simulink model "SMC_final"  (R2022b)
settings: Solver=ode14x  StartTime=0.0  StopTime=50  FixedStep=0.0002  RelTol=1e-3
undefined symbols (not defined in the file): g, I_xx, I_yy, I_zz, K_k_phi, K_k_psi, K_k_theta, K_k_x, K_k_y, K_k_z, lambda_phi, lambda_psi, lambda_theta, lambda_x, lambda_y, lambda_z, m, Psi_ref, X_ref, Y_ref, Z_ref
libraries: slpidlib x3
settings Model: Creator=User  LastModifiedBy=User
settings SolverCC: AlgebraicLoopSolver=TrustRegion
settings RTWCC: DLArmComputeVersion=19.05

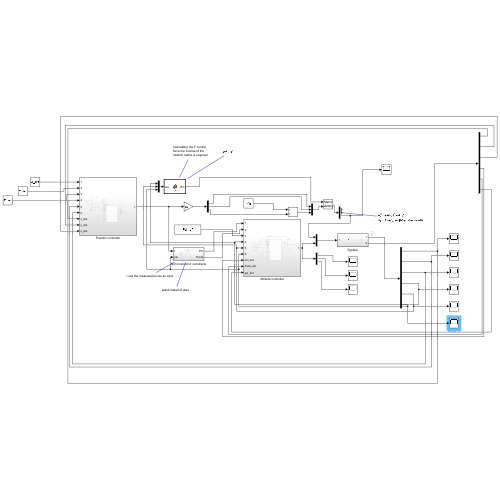
[thumbnail: Simulink's stored preview of the top-level diagram]
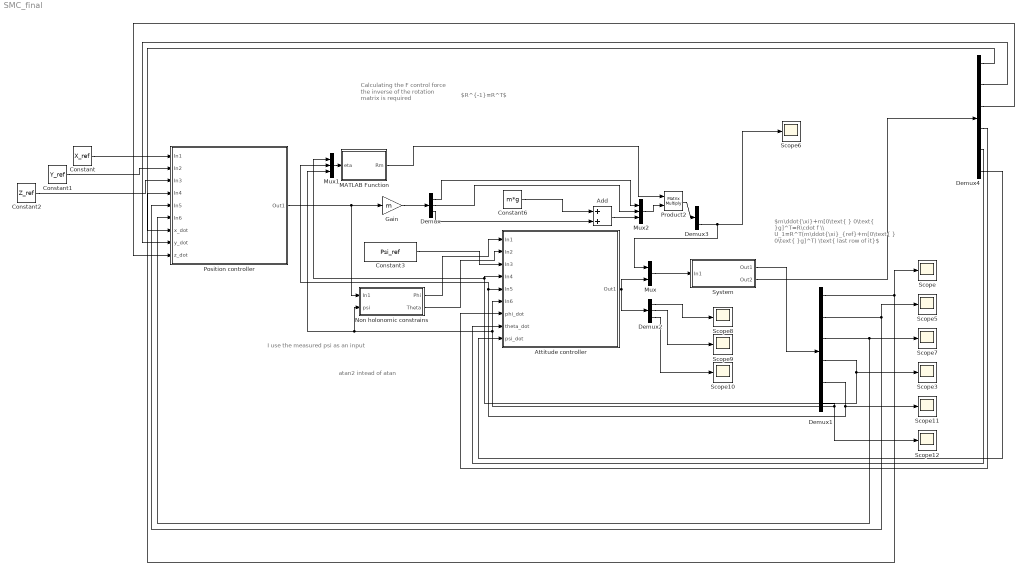
== system SMC_final ==
  note: $R^{-1}=R^T$
  note: $m\ddot{\xi}+m[0\text{ } 0\text{ }g]^T=R\cdot f \\ U_1=R^T(m\ddot{\xi}_{ref}+m[0\text{ } 0\text{ }g]^T) \text{ last row of it}$
  note: atan2 intead of atan
  note: Calculating the F control force the inverse of the rotation matrix is required
  note: I use the measured psi as an input
  Add : Sum
  Attitude controller : Subsystem
  Constant : Constant  Value=X_ref
  Constant1 : Constant  Value=Y_ref
  Constant2 : Constant  Value=Z_ref
  Constant3 : Constant  Value=Psi_ref
  Constant6 : Constant  Value=m*g
  Demux : Demux  Outputs=3
  Demux1 : Demux  Outputs=6
  Demux2 : Demux  Outputs=3
  Demux3 : Demux  Outputs=3
  Demux4 : Demux  Outputs=6
  Gain : Gain  Gain=m
  MATLAB Function : MATLAB Function  TreatAsAtomicUnit=on
  Mux : Mux  Inputs=2
  Mux1 : Mux  Inputs=3
  Mux2 : Mux  Inputs=3
  Non holonomic constrains : Subsystem
  Position controller : Subsystem
  Product2 : Product  Multiplication=Matrix(*)
  Scope{,3,5..12} (10 alike) : Scope
  System : Subsystem
  wires:
  System/1(Out1) -> Demux1/1
  Demux1/4 -> Scope3/1, Mux1/1, Attitude controller/4(In4)
  Demux1/1 -> Scope/1, Position controller/4(In4)
  Demux1/2 -> Scope5/1, Position controller/5(In5)
  Demux1/3 -> Scope7/1, Position controller/6(In6)
  Position controller/1(Out1) -> Non holonomic constrains/1(In1), Gain/1
  Non holonomic constrains/1(Phi) -> Attitude controller/1(In1)
  Non holonomic constrains/2(Theta) -> Attitude controller/2(In2)
  Demux1/5 -> Mux1/2, Attitude controller/5(In5), Scope11/1
  Demux1/6 -> Scope12/1, Non holonomic constrains/2(psi), Mux1/3, Attitude controller/6(In6)
  Attitude controller/1(Out1) -> Mux/2, Demux2/1
  Mux/1 -> System/1(In1)
  Demux/1 -> Mux2/1
  Demux/2 -> Mux2/2
  Demux2/1 -> Scope8/1
  Demux2/2 -> Scope9/1
  Demux2/3 -> Scope10/1
  Constant3/1 -> Attitude controller/3(In3)
  Demux/3 -> Add/2
  Mux1/1 -> MATLAB Function/1(eta)
  Add/1 -> Mux2/3
  MATLAB Function/1(Rm) -> Product2/1
  Mux2/1 -> Product2/2
  Product2/1 -> Demux3/1
  Demux3/3 -> Mux/1, Scope6/1
  Gain/1 -> Demux/1
  Constant/1 -> Position controller/1(In1)
  Constant1/1 -> Position controller/2(In2)
  Constant2/1 -> Position controller/3(In3)
  Constant6/1 -> Add/1
  System/2(Out2) -> Demux4/1
  Demux4/1 -> Position controller/7(x_dot)
  Demux4/2 -> Position controller/8(y_dot)
  Demux4/3 -> Position controller/9(z_dot)
  Demux4/4 -> Attitude controller/7(phi_dot)
  Demux4/5 -> Attitude controller/8(theta_dot)
  Demux4/6 -> Attitude controller/9(psi_dot)

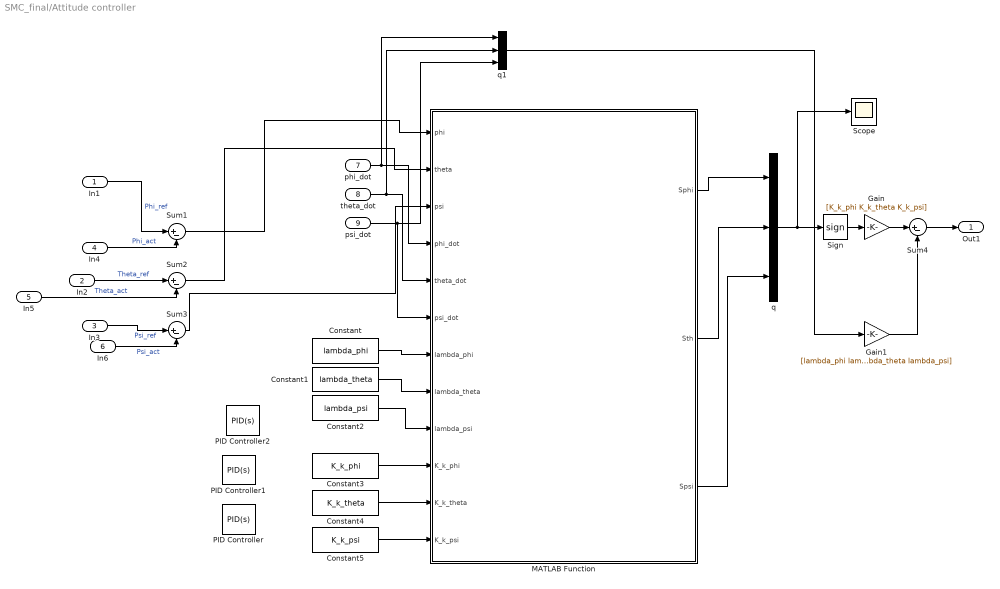
== system SMC_final/Attitude controller ==
  In1 : Inport
  In2 : Inport  Port=2
  In3 : Inport  Port=3
  In4 : Inport  Port=4
  In5 : Inport  Port=5
  In6 : Inport  Port=6
  phi_dot : Inport  Port=7
  theta_dot : Inport  Port=8
  psi_dot : Inport  Port=9
  Constant : Constant  Value=lambda_phi
  Constant1 : Constant  Value=lambda_theta
  Constant2 : Constant  Value=lambda_psi
  Constant3 : Constant  Value=K_k_phi
  Constant4 : Constant  Value=K_k_theta
  Constant5 : Constant  Value=K_k_psi
  Gain : Gain  Gain=[K_k_phi K_k_theta K_k_psi]
  Gain1 : Gain  Gain=[lambda_phi lambda_theta lambda_psi]
  MATLAB Function : MATLAB Function  TreatAsAtomicUnit=on
  PID Controller : slpidlib/PID Controller  Controller=PID  Form=Parallel  TimeDomain=Continuous-time  UseExternalTs=off  SampleTime=-1  IntegratorMethod=Forward Euler  FilterMethod=Forward Euler  ControllerParametersSource=internal  P=0.1  I=0  UseKiTs=off  D=0.05  N=100  UseFilter=on  TunerSelectOption=Transfer Function Based (PID Tuner App)  InitialConditionSource=internal  InitialConditionForIntegrator=0  InitialConditionForFilter=0  DifferentiatorICPrevScaledInput=0  ExternalReset=none  TrackingMode=off  Kt=1  LimitOutput=off  SatLimitsSource=internal  UpperSaturationLimit=inf  LowerSaturationLimit=-inf  LinearizeAsGain=on  AntiWindupMode=none  Kb=1  LimitIntegrator=off  UpperIntegratorSaturationLimit=inf  LowerIntegratorSaturationLimit=-inf  POutMin=[]  POutMax=[]  IOutMin=[]  IOutMax=[]  DOutMin=[]  DOutMax=[]  NOutMin=[]  NOutMax=[]  SumOutMin=[]  SumOutMax=[]  SaturationOutMin=[]  SaturationOutMax=[]  PParamMin=[]  PParamMax=[]  IParamMin=[]  IParamMax=[]  DParamMin=[]  DParamMax=[]  NParamMin=[]  NParamMax=[]  KbParamMin=[]  KbParamMax=[]  KtParamMin=[]  KtParamMax=[]  KbOutMin=[]  KbOutMax=[]  KtOutMin=[]  KtOutMax=[]  IntegratorOutMin=[]  IntegratorOutMax=[]  FilterOutMin=[]  FilterOutMax=[]  SumI1OutMin=[]  SumI1OutMax=[]  SumI2OutMin=[]  SumI2OutMax=[]  SumI3OutMin=[]  SumI3OutMax=[]  SumI4OutMin=[]  SumI4OutMax=[]  SumDOutMin=[]  SumDOutMax=[]  DifferentiatorOutMin=[]  DifferentiatorOutMax=[]  FilterDiffOutCoefMin=[]  FilterDiffOutCoefMax=[]  ReciprocalOutMin=[]  ReciprocalOutMax=[]  SumDenOutMin=[]  SumDenOutMax=[]  SumNumOutMin=[]  SumNumOutMax=[]  DivideOutMin=[]  DivideOutMax=[]  UdiffTsProdOutMin=[]  UdiffTsProdOutMax=[]  NTsProdOutMin=[]  NTsProdOutMax=[]  UintegralTsProdOutMin=[]  UintegralTsProdOutMax=[]  UngainTsProdOutMin=[]  UngainTsProdOutMax=[]  ClampingZeroOutDataTypeStr=Inherit: Inherit via back propagation  ClampingZeroOutMin=[]  ClampingZeroOutMax=[]  FilterDenConstantOutDataTypeStr=Inherit: Inherit via back propagation  FilterDenConstantOutMin=[]  FilterDenConstantOutMax=[]  PCopyOutDataTypeStr=Inherit: Inherit via back propagation  PCopyOutMin=[]  PCopyOutMax=[]  NCopyOutDataTypeStr=Inherit: Inherit via back propagation  NCopyOutMin=[]  NCopyOutMax=[]  IntegratorContinuousStateAttributes=''  IntegratorStateMustResolveToSignalObject=off  IntegratorRTWStateStorageClass=Auto  FilterContinuousStateAttributes=''  FilterStateMustResolveToSignalObject=off  FilterRTWStateStorageClass=Auto  ParallelPVariant=InternalParameters  IdealPVariant=Disabled  IVariant=InternalParameters  DVariant=InternalParameters  IntegratorVariant=Continuous  SatVariant=Disabled  AWVariant=Passthrough  PCopyVariant=Disabled  TRVariant=Disabled  FdbkBlocksVariant=Forward  IdealPFdbkVariant=Disabled  SatFdbkVariant=Disabled  DerivativeFilterVariant=ContFilter  NVariant=InternalParameters  NCopyVariant=Disabled  FilterICVariant=InternalICsFilter  IntegratorICVariant=InternalICs  ExternalResetVariant=Disabled  TRSumVariant=Passthrough  SumFdbkVariant=Disabled  SumVariant=Sum_PID  TsampFilterVariant=InternalTs  TsampNgainVariant=Passthrough  TsampIntegralVariant=Passthrough  ExternalSaturationOutDataTypeStr=Inherit: Same as second input
  PID Controller1 : slpidlib/PID Controller  Controller=PID  Form=Parallel  TimeDomain=Continuous-time  UseExternalTs=off  SampleTime=-1  IntegratorMethod=Forward Euler  FilterMethod=Forward Euler  ControllerParametersSource=internal  P=0.1  I=0  UseKiTs=off  D=0.05  N=100  UseFilter=on  TunerSelectOption=Transfer Function Based (PID Tuner App)  InitialConditionSource=internal  InitialConditionForIntegrator=0  InitialConditionForFilter=0  DifferentiatorICPrevScaledInput=0  ExternalReset=none  TrackingMode=off  Kt=1  LimitOutput=off  SatLimitsSource=internal  UpperSaturationLimit=inf  LowerSaturationLimit=-inf  LinearizeAsGain=on  AntiWindupMode=none  Kb=1  LimitIntegrator=off  UpperIntegratorSaturationLimit=inf  LowerIntegratorSaturationLimit=-inf  POutMin=[]  POutMax=[]  IOutMin=[]  IOutMax=[]  DOutMin=[]  DOutMax=[]  NOutMin=[]  NOutMax=[]  SumOutMin=[]  SumOutMax=[]  SaturationOutMin=[]  SaturationOutMax=[]  PParamMin=[]  PParamMax=[]  IParamMin=[]  IParamMax=[]  DParamMin=[]  DParamMax=[]  NParamMin=[]  NParamMax=[]  KbParamMin=[]  KbParamMax=[]  KtParamMin=[]  KtParamMax=[]  KbOutMin=[]  KbOutMax=[]  KtOutMin=[]  KtOutMax=[]  IntegratorOutMin=[]  IntegratorOutMax=[]  FilterOutMin=[]  FilterOutMax=[]  SumI1OutMin=[]  SumI1OutMax=[]  SumI2OutMin=[]  SumI2OutMax=[]  SumI3OutMin=[]  SumI3OutMax=[]  SumI4OutMin=[]  SumI4OutMax=[]  SumDOutMin=[]  SumDOutMax=[]  DifferentiatorOutMin=[]  DifferentiatorOutMax=[]  FilterDiffOutCoefMin=[]  FilterDiffOutCoefMax=[]  ReciprocalOutMin=[]  ReciprocalOutMax=[]  SumDenOutMin=[]  SumDenOutMax=[]  SumNumOutMin=[]  SumNumOutMax=[]  DivideOutMin=[]  DivideOutMax=[]  UdiffTsProdOutMin=[]  UdiffTsProdOutMax=[]  NTsProdOutMin=[]  NTsProdOutMax=[]  UintegralTsProdOutMin=[]  UintegralTsProdOutMax=[]  UngainTsProdOutMin=[]  UngainTsProdOutMax=[]  ClampingZeroOutDataTypeStr=Inherit: Inherit via back propagation  ClampingZeroOutMin=[]  ClampingZeroOutMax=[]  FilterDenConstantOutDataTypeStr=Inherit: Inherit via back propagation  FilterDenConstantOutMin=[]  FilterDenConstantOutMax=[]  PCopyOutDataTypeStr=Inherit: Inherit via back propagation  PCopyOutMin=[]  PCopyOutMax=[]  NCopyOutDataTypeStr=Inherit: Inherit via back propagation  NCopyOutMin=[]  NCopyOutMax=[]  IntegratorContinuousStateAttributes=''  IntegratorStateMustResolveToSignalObject=off  IntegratorRTWStateStorageClass=Auto  FilterContinuousStateAttributes=''  FilterStateMustResolveToSignalObject=off  FilterRTWStateStorageClass=Auto  ParallelPVariant=InternalParameters  IdealPVariant=Disabled  IVariant=InternalParameters  DVariant=InternalParameters  IntegratorVariant=Continuous  SatVariant=Disabled  AWVariant=Passthrough  PCopyVariant=Disabled  TRVariant=Disabled  FdbkBlocksVariant=Forward  IdealPFdbkVariant=Disabled  SatFdbkVariant=Disabled  DerivativeFilterVariant=ContFilter  NVariant=InternalParameters  NCopyVariant=Disabled  FilterICVariant=InternalICsFilter  IntegratorICVariant=InternalICs  ExternalResetVariant=Disabled  TRSumVariant=Passthrough  SumFdbkVariant=Disabled  SumVariant=Sum_PID  TsampFilterVariant=InternalTs  TsampNgainVariant=Passthrough  TsampIntegralVariant=Passthrough  ExternalSaturationOutDataTypeStr=Inherit: Same as second input
  PID Controller2 : slpidlib/PID Controller  Controller=PID  Form=Parallel  TimeDomain=Continuous-time  UseExternalTs=off  SampleTime=-1  IntegratorMethod=Forward Euler  FilterMethod=Forward Euler  ControllerParametersSource=internal  P=0.1  I=0  UseKiTs=off  D=0.15  N=100  UseFilter=on  TunerSelectOption=Transfer Function Based (PID Tuner App)  InitialConditionSource=internal  InitialConditionForIntegrator=0  InitialConditionForFilter=0  DifferentiatorICPrevScaledInput=0  ExternalReset=none  TrackingMode=off  Kt=1  LimitOutput=off  SatLimitsSource=internal  UpperSaturationLimit=inf  LowerSaturationLimit=-inf  LinearizeAsGain=on  AntiWindupMode=none  Kb=1  LimitIntegrator=off  UpperIntegratorSaturationLimit=inf  LowerIntegratorSaturationLimit=-inf  POutMin=[]  POutMax=[]  IOutMin=[]  IOutMax=[]  DOutMin=[]  DOutMax=[]  NOutMin=[]  NOutMax=[]  SumOutMin=[]  SumOutMax=[]  SaturationOutMin=[]  SaturationOutMax=[]  PParamMin=[]  PParamMax=[]  IParamMin=[]  IParamMax=[]  DParamMin=[]  DParamMax=[]  NParamMin=[]  NParamMax=[]  KbParamMin=[]  KbParamMax=[]  KtParamMin=[]  KtParamMax=[]  KbOutMin=[]  KbOutMax=[]  KtOutMin=[]  KtOutMax=[]  IntegratorOutMin=[]  IntegratorOutMax=[]  FilterOutMin=[]  FilterOutMax=[]  SumI1OutMin=[]  SumI1OutMax=[]  SumI2OutMin=[]  SumI2OutMax=[]  SumI3OutMin=[]  SumI3OutMax=[]  SumI4OutMin=[]  SumI4OutMax=[]  SumDOutMin=[]  SumDOutMax=[]  DifferentiatorOutMin=[]  DifferentiatorOutMax=[]  FilterDiffOutCoefMin=[]  FilterDiffOutCoefMax=[]  ReciprocalOutMin=[]  ReciprocalOutMax=[]  SumDenOutMin=[]  SumDenOutMax=[]  SumNumOutMin=[]  SumNumOutMax=[]  DivideOutMin=[]  DivideOutMax=[]  UdiffTsProdOutMin=[]  UdiffTsProdOutMax=[]  NTsProdOutMin=[]  NTsProdOutMax=[]  UintegralTsProdOutMin=[]  UintegralTsProdOutMax=[]  UngainTsProdOutMin=[]  UngainTsProdOutMax=[]  ClampingZeroOutDataTypeStr=Inherit: Inherit via back propagation  ClampingZeroOutMin=[]  ClampingZeroOutMax=[]  FilterDenConstantOutDataTypeStr=Inherit: Inherit via back propagation  FilterDenConstantOutMin=[]  FilterDenConstantOutMax=[]  PCopyOutDataTypeStr=Inherit: Inherit via back propagation  PCopyOutMin=[]  PCopyOutMax=[]  NCopyOutDataTypeStr=Inherit: Inherit via back propagation  NCopyOutMin=[]  NCopyOutMax=[]  IntegratorContinuousStateAttributes=''  IntegratorStateMustResolveToSignalObject=off  IntegratorRTWStateStorageClass=Auto  FilterContinuousStateAttributes=''  FilterStateMustResolveToSignalObject=off  FilterRTWStateStorageClass=Auto  ParallelPVariant=InternalParameters  IdealPVariant=Disabled  IVariant=InternalParameters  DVariant=InternalParameters  IntegratorVariant=Continuous  SatVariant=Disabled  AWVariant=Passthrough  PCopyVariant=Disabled  TRVariant=Disabled  FdbkBlocksVariant=Forward  IdealPFdbkVariant=Disabled  SatFdbkVariant=Disabled  DerivativeFilterVariant=ContFilter  NVariant=InternalParameters  NCopyVariant=Disabled  FilterICVariant=InternalICsFilter  IntegratorICVariant=InternalICs  ExternalResetVariant=Disabled  TRSumVariant=Passthrough  SumFdbkVariant=Disabled  SumVariant=Sum_PID  TsampFilterVariant=InternalTs  TsampNgainVariant=Passthrough  TsampIntegralVariant=Passthrough  ExternalSaturationOutDataTypeStr=Inherit: Same as second input
  Scope : Scope
  Sign : Signum  ZeroCross=off
  Sum{1..4} (4 alike) : Sum  Inputs=|+-
  q : Mux  Inputs=3
  q1 : Mux  Inputs=3
  Out1 : Outport
  wires:
  In1/1 -> Sum1/1  "Phi_ref"
  In4/1 -> Sum1/2  "Phi_act"
  In2/1 -> Sum2/1  "Theta_ref"
  In5/1 -> Sum2/2  "Theta_act"
  In3/1 -> Sum3/1  "Psi_ref"
  In6/1 -> Sum3/2  "Psi_act"
  MATLAB Function/2(Sth) -> q/2
  MATLAB Function/1(Sphi) -> q/1
  MATLAB Function/3(Spsi) -> q/3
  Sum1/1 -> MATLAB Function/1(phi)
  Sum2/1 -> MATLAB Function/2(theta)
  Sum3/1 -> MATLAB Function/3(psi)
  phi_dot/1 -> q1/1, MATLAB Function/4(phi_dot)
  theta_dot/1 -> q1/2, MATLAB Function/5(theta_dot)
  psi_dot/1 -> q1/3, MATLAB Function/6(psi_dot)
  Constant/1 -> MATLAB Function/7(lambda_phi)
  Constant1/1 -> MATLAB Function/8(lambda_theta)
  Constant2/1 -> MATLAB Function/9(lambda_psi)
  Constant3/1 -> MATLAB Function/10(K_k_phi)
  Constant5/1 -> MATLAB Function/12(K_k_psi)
  Constant4/1 -> MATLAB Function/11(K_k_theta)
  Sum4/1 -> Out1/1
  q/1 -> Scope/1, Sign/1
  Sign/1 -> Gain/1
  Gain/1 -> Sum4/1
  q1/1 -> Gain1/1
  Gain1/1 -> Sum4/2

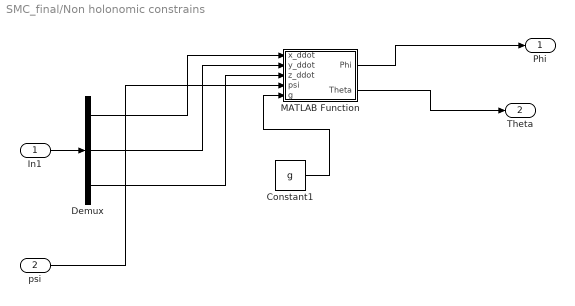
== system SMC_final/Non holonomic constrains ==
  In1 : Inport
  psi : Inport  Port=2
  Constant1 : Constant  Value=g
  Demux : Demux  Outputs=3
  MATLAB Function : MATLAB Function  TreatAsAtomicUnit=on
  Phi : Outport
  Theta : Outport  Port=2
  wires:
  In1/1 -> Demux/1
  Demux/1 -> MATLAB Function/1(x_ddot)
  Demux/2 -> MATLAB Function/2(y_ddot)
  Demux/3 -> MATLAB Function/3(z_ddot)
  Constant1/1 -> MATLAB Function/5(g)
  MATLAB Function/1(Phi) -> Phi/1
  MATLAB Function/2(Theta) -> Theta/1
  psi/1 -> MATLAB Function/4(psi)

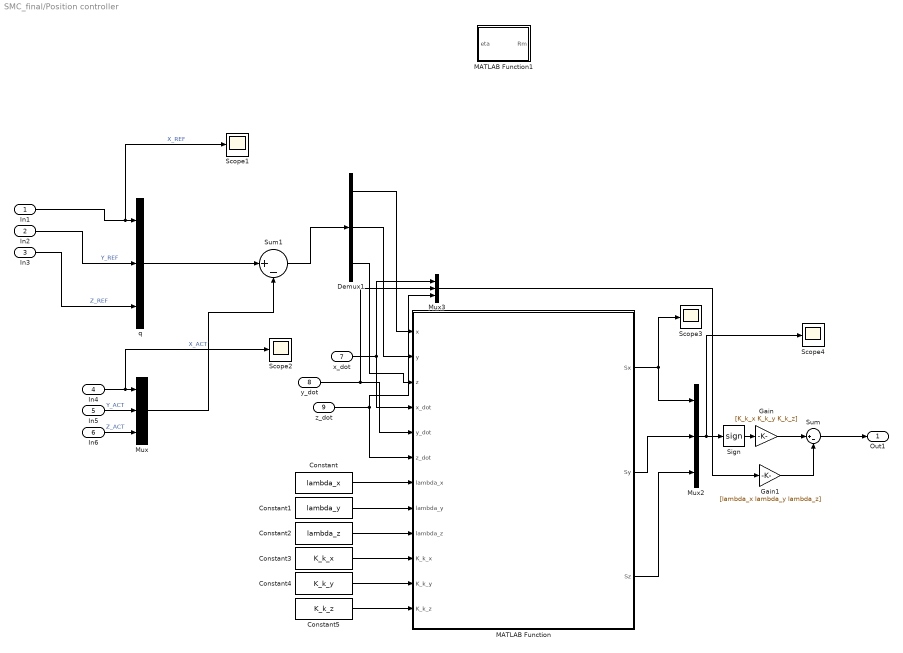
== system SMC_final/Position controller ==
  In1 : Inport
  In2 : Inport  Port=2
  In3 : Inport  Port=3
  In4 : Inport  Port=4
  In5 : Inport  Port=5
  In6 : Inport  Port=6
  x_dot : Inport  Port=7
  y_dot : Inport  Port=8
  z_dot : Inport  Port=9
  Constant : Constant  Value=lambda_x
  Constant1 : Constant  Value=lambda_y
  Constant2 : Constant  Value=lambda_z
  Constant3 : Constant  Value=K_k_x
  Constant4 : Constant  Value=K_k_y
  Constant5 : Constant  Value=K_k_z
  Demux1 : Demux  Outputs=3
  Gain : Gain  Gain=[K_k_x K_k_y K_k_z]
  Gain1 : Gain  Gain=[lambda_x lambda_y lambda_z]
  MATLAB Function : MATLAB Function  TreatAsAtomicUnit=on
  MATLAB Function1 : MATLAB Function  TreatAsAtomicUnit=on
  Mux : Mux  Inputs=3
  Mux2 : Mux  Inputs=3
  Mux3 : Mux  Inputs=3
  Scope{1..4} (4 alike) : Scope
  Sign : Signum  ZeroCross=off
  Sum : Sum  Inputs=|+-
  Sum1 : Sum  Inputs=|+-
  q : Mux  Inputs=3
  Out1 : Outport
  wires:
  In3/1 -> q/3  "Z_REF"
  In2/1 -> q/2  "Y_REF"
  In1/1 -> Scope1/1, q/1  "X_REF"
  In4/1 -> Scope2/1, Mux/1  "X_ACT"
  In5/1 -> Mux/2  "Y_ACT"
  In6/1 -> Mux/3  "Z_ACT"
  q/1 -> Sum1/1
  Mux/1 -> Sum1/2
  Sum1/1 -> Demux1/1
  MATLAB Function/2(Sy) -> Mux2/2
  MATLAB Function/1(Sx) -> Scope3/1, Mux2/1
  MATLAB Function/3(Sz) -> Mux2/3
  y_dot/1 -> Mux3/2, MATLAB Function/5(y_dot)
  z_dot/1 -> Mux3/3, MATLAB Function/6(z_dot)
  x_dot/1 -> Mux3/1, MATLAB Function/4(x_dot)
  Demux1/1 -> MATLAB Function/1(x)
  Demux1/2 -> MATLAB Function/2(y)
  Demux1/3 -> MATLAB Function/3(z)
  Constant/1 -> MATLAB Function/7(lambda_x)
  Constant1/1 -> MATLAB Function/8(lambda_y)
  Constant2/1 -> MATLAB Function/9(lambda_z)
  Constant3/1 -> MATLAB Function/10(K_k_x)
  Constant4/1 -> MATLAB Function/11(K_k_y)
  Constant5/1 -> MATLAB Function/12(K_k_z)
  Mux2/1 -> Scope4/1, Sign/1
  Sign/1 -> Gain/1
  Gain/1 -> Sum/1
  Mux3/1 -> Gain1/1
  Gain1/1 -> Sum/2
  Sum/1 -> Out1/1

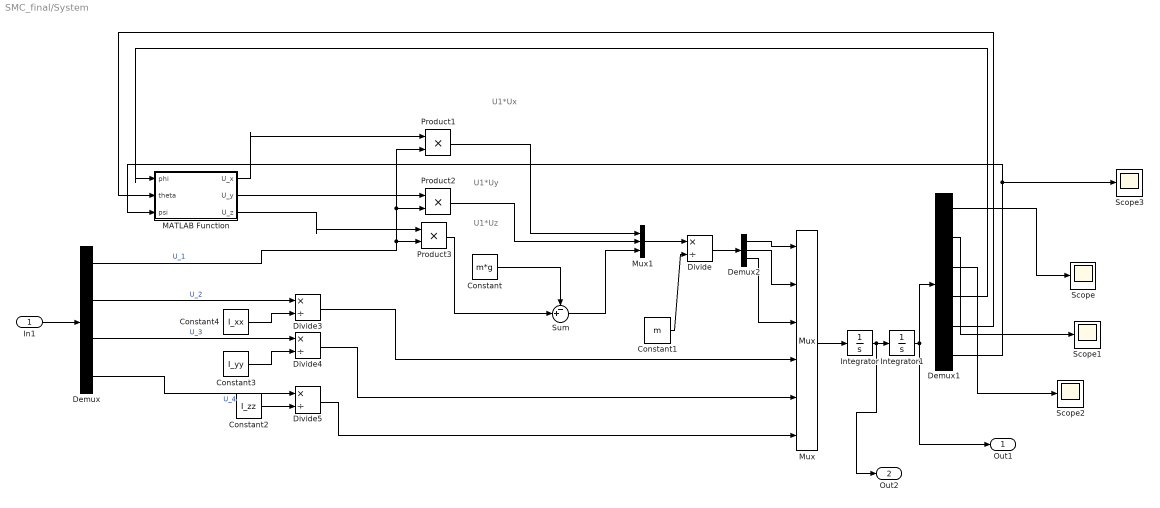
== system SMC_final/System ==
  note: U1*Ux
  note: U1*Uy
  note: U1*Uz
  In1 : Inport
  Constant : Constant  Value=m*g
  Constant1 : Constant  Value=m
  Constant2 : Constant  Value=I_zz
  Constant3 : Constant  Value=I_yy
  Constant4 : Constant  Value=I_xx
  Demux : Demux
  Demux1 : Demux  Outputs=6
  Demux2 : Demux  Outputs=3
  Divide{,3..5} (4 alike) : Product  Inputs=*/
  Integrator : Integrator
  Integrator1 : Integrator
  MATLAB Function : MATLAB Function  TreatAsAtomicUnit=on
  Mux : Mux  Inputs=6
  Mux1 : Mux  Inputs=3
  Product1 : Product
  Product2 : Product
  Product3 : Product
  Scope{,1..3} (4 alike) : Scope
  Sum : Sum  Inputs=-+|
  Out1 : Outport
  Out2 : Outport  Port=2
  wires:
  In1/1 -> Demux/1
  Mux/1 -> Integrator/1
  Integrator/1 -> Out2/1, Integrator1/1
  MATLAB Function/1(U_x) -> Product1/1
  MATLAB Function/2(U_y) -> Product2/1
  Demux/1 -> Product1/2, Product2/2, Product3/2  "U_1"
  Integrator1/1 -> Demux1/1, Out1/1
  Demux1/4 -> MATLAB Function/1(phi)
  Demux1/5 -> MATLAB Function/2(theta)
  Demux1/6 -> Scope3/1, MATLAB Function/3(psi)
  Demux1/1 -> Scope/1
  Demux1/2 -> Scope1/1
  Demux1/3 -> Scope2/1
  Demux/2 -> Divide3/1  "U_2"
  Constant4/1 -> Divide3/2
  Demux/3 -> Divide4/1  "U_3"
  Demux/4 -> Divide5/1  "U_4"
  Constant3/1 -> Divide4/2
  Constant2/1 -> Divide5/2
  Divide3/1 -> Mux/4
  Divide4/1 -> Mux/5
  Divide5/1 -> Mux/6
  MATLAB Function/3(U_z) -> Product3/1
  Product3/1 -> Sum/2
  Constant/1 -> Sum/1
  Product1/1 -> Mux1/1
  Product2/1 -> Mux1/2
  Sum/1 -> Mux1/3
  Mux1/1 -> Divide/1
  Constant1/1 -> Divide/2
  Divide/1 -> Demux2/1
  Demux2/1 -> Mux/1
  Demux2/2 -> Mux/2
  Demux2/3 -> Mux/3

== matlab function SMC_final/Non holonomic constrains/MATLAB Function ==
  data: x_ddot input; Phi output; y_ddot input; z_ddot input; psi input; Theta output; g input
function [Phi, Theta] = fcn(x_ddot,y_ddot,z_ddot,psi,g)


Phi = asin((x_ddot*sin(psi)-y_ddot*cos(psi))/(sqrt(x_ddot^2+y_ddot^2+(z_ddot+g)^2)));
Theta =atan2((x_ddot*cos(psi )+y_ddot*sin(psi)),(z_ddot+g));

== matlab function SMC_final/System/MATLAB Function ==
  data: phi input; U_x output; theta input; psi input; U_y output; U_z output
function [U_x,U_y,U_z] = fcn(phi,theta,psi)


U_x = cos(phi)*sin(theta)*cos(psi)+sin(phi)*sin(psi);
U_y = cos(phi)*sin(theta)*sin(psi)-sin(phi)*cos(psi);
U_z =cos(phi)*cos(theta);

== matlab function SMC_final/Position controller/MATLAB Function1 ==
  data: eta input size=3; Rm output
function Rm = R(eta)

phi = eta(1);
theta = eta(2);
psi = eta(3);

Rx = [1 0 0; 0 cos(phi) -sin(phi); 0 sin(phi) cos(phi)];
Ry = [cos(theta) 0 sin(theta); 0 1 0; -sin(theta) 0 cos(theta)];
Rz = [cos(psi) -sin(psi) 0; sin(psi) cos(psi) 0; 0 0 1];
Rm = (Rz*Ry*Rx)';

== matlab function SMC_final/MATLAB Function ==
  data: eta input size=3; Rm output
function Rm = R(eta)

phi = eta(1);
theta = eta(2);
psi = eta(3);

Rx = [1 0 0; 0 cos(phi) -sin(phi); 0 sin(phi) cos(phi)];
Ry = [cos(theta) 0 sin(theta); 0 1 0; -sin(theta) 0 cos(theta)];
Rz = [cos(psi) -sin(psi) 0; sin(psi) cos(psi) 0; 0 0 1];
Rm = (Rz*Ry*Rx)';

== matlab function SMC_final/Position controller/MATLAB Function ==
  data: x input; Sx output; y input; z input; x_dot input; Sy output; y_dot input; z_dot input; Sz output; lambda_x input; lambda_y input; lambda_z input; K_k_x input; K_k_y input; K_k_z input
function [Sx,Sy,Sz] = fcn(x,y,z,x_dot,y_dot,z_dot,lambda_x,lambda_y,lambda_z,K_k_x,K_k_y,K_k_z)



Sx=(-x_dot+lambda_x*x);
Sy=(-y_dot+lambda_y*y);
Sz=(-z_dot+lambda_z*z);

== matlab function SMC_final/Attitude controller/MATLAB Function ==
  data: phi input; Sphi output; theta input; psi input; phi_dot input; Sth output; theta_dot input; psi_dot input; lambda_phi input; lambda_theta input; lambda_psi input; K_k_phi input; K_k_theta input; K_k_psi input; Spsi output
function [Sphi,Sth,Spsi] = fcn(phi,theta,psi,phi_dot,theta_dot,psi_dot,lambda_phi,lambda_theta,lambda_psi,K_k_phi,K_k_theta,K_k_psi)



Sphi=(-phi_dot+lambda_phi*phi);
Sth=(-theta_dot+lambda_theta*theta);
Spsi=(-psi_dot+lambda_psi*psi);
